simulink library "SUB_ECU_L4_MABX_HW_Interface_PIC_KW"  (R2018a)
settings: Solver=VariableStepAuto  StartTime=0.0  StopTime=10.0  RelTol=1e-3
PostLoadFcn:
  | , if any(exist('dsrtsu_mdlpostloadfcn', 'file') == [2, 3, 6]), try dsrtsu_mdlpostloadfcn('Execute', bdroot); catch fprintf('Error in PostLoadFcn (dsrtsu_mdlpostloadfcn) for model "%s":\n %s\n', bdroot, lasterr); end, end,
undefined symbols (not defined in the file or in its folder): CANR_PROPB_REAX_3_13_CHANNEL_APV, CANR_PROPB_REAX_4_13_CHANNEL_APV, CANR_PROPB_XPR_1_50_CHANNEL_APV, ENUM_CAN_RX_T, ENUM_CAN_TX_T, ENUM_REAX_OPERATION_MODE_T, ENUM_SIGNAL_HEALTH_T, ENUM_XBR_CONTROL_MODE_T, ENUM_XBR_EBI_MODE_T, ENUM_XBR_PASS_THROUGH_ACTIVE_T, ENUM_XBR_PRIORITY_T, ENUM_XPR_INHIBIT_PARK_MANUAL_T, ENUM_XPR_INHIBIT_UNPARK_MANUAL_T, ENUM_XPR_PARK_MANUAL_T, ENUM_XPR_UNPARK_MANUAL_T, PROPB_REAX_1_E4_DES_POS_SIG_SRC_APV, PROPB_REAX_1_E4_DESIRED_OPMODE_APV, PROPB_REAX_1_E4_DESIRED_POSITION_APV, PROPB_REAX_CHANNEL_APV, ptc_matlab_lib
libraries: PTC_MBDS_LIB x292, rtican x158, simulink x58, EmE_MBD_Blockset x38, rti1401lib_dio_type4 x13, simulink_need_slupdate x7, rti1401lib_adc_type4 x3, rtmapslib x3, $bdroot x3, dsa_tcpip_lib x2, SUB_ECU_L4_MABX_HW_Interface_PTC_1571 x1, rtitasklib x1
(part 13 of 48)

== system SUB_ECU_L4_MABX_HW_Interface_PIC_KW/CAN_PIC_KW/CAN_RX_EEC1_00/RX_CAN_1 ==
  Enable : Inport
  Bus Creator3 : BusCreator  Inputs=11
  Data Type Conversion10 : DataTypeConversion  OutDataTypeStr=double  SaturateOnIntegerOverflow=on
  Data Type Conversion8 : DataTypeConversion  OutDataTypeStr=boolean  SaturateOnIntegerOverflow=on
  Data Type Conversion9 : DataTypeConversion  OutDataTypeStr=double  SaturateOnIntegerOverflow=on
  EEC1_001 : rtican/RTICAN Receive (RX)   Reserved1=[]  Reserved2=[]  Reserved3=[]  Reserved4=[]  SfcnMessage=[]  Msg_Struct=[]  BoardTypeNo=[]  BoardNo=[]  ChannelNo=[]  Parameters=[]  DialogFcn=[]  UnitName=[]  Revision=[]  UnitValues=[]  DSProperties=struct('RTI',struct('Version',uint32(5),'BlockType',struct('isSLSource',uint8(1),'isSLSink',uint8(1),'isHWSource',uint8(0),'isHWSink',uint8(0),'isSetup',uint8(0),'isInline',uint8(1),'isNonInline',uint8(0),'isInterrupt',uint8(0),'isChannelwise',uint8(0)),'IOBoardType','RTICAN','UnitType','MESSAGE','Identifier','RX','DialogType','MSVC','BlockSet','RTICAN','SlaveProcessor','CAN'))  RTIBlockInterface=struct('OutputPortsWidth',int32([1 1 1 1 1 1 1 1 1 1 1]),'OutputPortsActive',ones(1,11),'OutputPortsName',{{'EngTorqueMode','ActlEngPrcntTrqueHighResolution','DriversDemandEngPercentTorque','ActualEngPercentTorque','EngSpeed','SrcAddrssOfCtrllngDvcFrEngCntrl','EngStarterMode','EngDemandPercentTorque',['RX status'],['RX time'],['RX delta time']}},'OutputPortsDataType',{{'SS_DOUBLE','SS_DOUBLE','SS_DOUBLE','SS_DOUBLE','SS_DOUBLE','SS_DOUBLE','SS_DOUBLE','SS_DOUBLE','SS_DOUBLE','SS_DOUBLE','SS_DOUBLE'}},'OutputPortsLabel',{{'EngTorqueMode','ActlEngPrcntTrqueHighResolution','DriversDemandEngPercentTorque','ActualEngPercentTorque','EngSpeed','SrcAddrssOfCtrllngDvcFrEngCntrl','EngStarterMode','EngDemandPercentTorque','','',''}},'OutputPortsLabelMode','ON','InputPortsWidth',int32(0),'InputPortsActive',0,'DialogFcn','rtican_message_interface_gui','BlockDisplay',{{'','center'}},'IconTransparency','on','ParameterTunableNames',{{}},'InitLevel',3,'BlockName',struct('Token',{{'EEC1_00'}}),'SampleTime',{{-1}},'TriggerPort',{{'none'}},'EnablePort',{{'yes'}})  RTIBlockParameters=struct('BoardTypeNo',{{1,'OFF',[]}},'BoardNo',{{1,'ON',[1 16]}},'ChannelNo',{{1,'ON',[1 2]}},'Parameters',{{struct('DataFileSupport',struct('DataFileSelectedMaster',1,'DataFileSelectedLocal',1,'DataFileName','c:\localdata\chris\advanced_tech\adas\level4_rcp\truck1571\dbc\j1939_famosdbcwithfusion.dbc|','DataFileDate',{{{['03-Apr-2017 12:55:40']}}},'SelectedFile','dbc\j1939_famosdbcwithfusion.dbc'),'Options',struct('StatusSelected',1,'TimeSelected',1,'DeltaTimeSelected',1,'BytePortSelected',0,'MessageLengthSelected',0,'TriggerPort',struct('Selected',0,'TriggerType',0),'UserCoding',struct('Selected',0,'InterfaceFile','UserDecodingFile','FcnName','UserDecodeFcn','InportSelected',0,'InportWidth',1,'OutportSelected',0,'OutportWidth',1),'EnablePortSelected',1,'SignalOnPortnameSelected',1,'UseRXService',1),'Message',struct('MsgOnBlocknameSelected',1,'MsgName','EEC1_00','MsgIdFormat',1,'MsgId',217056256,'MsgLength',8,'NumSignals',8,'SampleTime',-1,'Signal',struct('SgnName',{'EngTorqueMode','ActlEngPrcntTrqueHighResolution','DriversDemandEngPercentTorque','ActualEngPercentTorque','EngSpeed','SrcAddrssOfCtrllngDvcFrEngCntrl','EngStarterMode','EngDemandPercentTorque'},'SgnStartBit',{0,4,8,16,24,40,48,56},'SgnLength',{4,4,8,8,16,8,4,8},'SgnType',{0,0,0,0,0,0,0,0},'ModeValue',{-1,-1,-1,-1,-1,-1,-1,-1},'DataType',{0,0,0,0,0,0,0,0},'ByteLayout',{0,0,0,0,0,0,0,0},'Factor',{1,2^-3,1,1,2^-3,1,1,1},'Offset',{0,0,-125,-125,0,0,0,-125},'SgnComment',{{['State signal which indicates which engine torque mode is currently generating, limiting, or controlling the torque.']},{['This parameter displays an additional torque in percent of the reference engine torque.']},{['The requested torque output of the engine by the driver.']},{['The calculated output torque of the engine.']},{['Actual engine speed which is calculated over a minimum crankshaft angle of 720 degrees divided by the number of cylinders.']},{['The source address of the SAE J1939 device currently controlling the engine.']},{['There are several phases in a starting action and different reasons why a start cannot take place.']},{['The requested torque output of the engine by all dynamic internal inputs, including smoke control, noise control and low']}},'SgnUnit',{'','%','%','%','rpm','','','%'},'Min',{0,0,-125,-125,0,0,0,-125},'Max',{15,0.875,125,125,8031.875,255,15,125},'SLDataType',{'SS_DOUBLE','SS_DOUBLE','SS_DOUBLE','SS_DOUBLE','SS_DOUBLE','SS_DOUBLE','SS_DOUBLE','SS_DOUBLE'}),'MsgIdNumFormat',0,'MsgComment',{{['Electronic Engine Controller 1']}}),'Version',1.2,'general',struct('isFromLib',0)),'OFF',[]}},'GroupId',{{struct('Group',{{'RTICAN'}},'No',1,'Behavior',{{'NAMECHANGE'}},'BlockType',{{'SINK'}},'NameChangeFlag',0),'OFF',[]}},'SFcnRTICANMessage',{{struct('MsgType','RX','SFcnPortType','Scalar','MsgName','EEC1_00','MsgIdFormat','XTD','MsgId',217056256,'MsgLength',8,'NumSignals',8,'SampleTime',-1,'Signal',struct('SgnName',{'EngTorqueMode','ActlEngPrcntTrqueHighResolution','DriversDemandEngPercentTorque','ActualEngPercentTorque','EngSpeed','SrcAddrssOfCtrllngDvcFrEngCntrl','EngStarterMode','EngDemandPercentTorque'},'SgnStartBit',{0,4,8,16,24,40,48,56},'SgnLength',{4,4,8,8,16,8,4,8},'SgnType',{'standard','standard','standard','standard','standard','standard','standard','standard'},'ModeValue',{-1,-1,-1,-1,-1,-1,-1,-1},'DataType',{['unsigned int'],['unsigned int'],['unsigned int'],['unsigned int'],['unsigned int'],['unsigned int'],['unsigned int'],['unsigned int']},'ByteLayout',{['little endian'],['little endian'],['little endian'],['little endian'],['little endian'],['little endian'],['little endian'],['little endian']},'Factor',{1,2^-3,1,1,2^-3,1,1,1},'Offset',{0,0,-125,-125,0,0,0,-125},'SLDataType',{'SS_DOUBLE','SS_DOUBLE','SS_DOUBLE','SS_DOUBLE','SS_DOUBLE','SS_DOUBLE','SS_DOUBLE','SS_DOUBLE'}),'StatusSelected','yes','TimeSelected','yes','DeltaTimeSelected','yes','BytePortSelected','no','MessageLengthSelected','no','TriggerPort',struct('Selected','no','TriggerType',0),'UserCoding',struct('Selected','no','InterfaceFile','UserDecodingFile','FcnName','UserDecodeFcn','InportSelected','no','InportWidth',1,'OutportSelected','no','OutportWidth',1),'EnablePortSelected','yes','UseRXService','yes','BoardType','DS1','BoardNo',1,'ControllerNo',1),'OFF',[]}},'TLCFileName',{{'rtican_rx_message','OFF',[]}})  RTISFcnParameters=struct('SFcnRTICANMessage','struct','TLCFileName','char')  RTIBlockParaDefault=struct('BoardTypeNo',4302,'BoardNo',1,'ChannelNo',1,'Parameters',struct('DataFileSupport',struct('DataFileSelectedMaster',0,'DataFileSelectedLocal',0,'DataFileName','','DataFileDate','','SelectedFile',['<no file selected>']),'Options',struct('StatusSelected',1,'TimeSelected',1,'DeltaTimeSelected',1,'BytePortSelected',0,'MessageLengthSelected',0,'TriggerPort',struct('Selected',0,'TriggerType','rising'),'UserCoding',struct('Selected',0,'InterfaceFile','UserDecodingFile','FcnName','UserDecodeFcn','InportSelected',0,'InportWidth',1,'OutportSelected',0,'OutportWidth',1),'EnablePortSelected',0,'SignalOnPortnameSelected',1,'UseRXService',0),'Message',struct('MsgOnBlocknameSelected',0,'MsgName',['RX Message'],'MsgIdFormat',0,'MsgId',100,'MsgLength',8,'NumSignals',1,'SampleTime',-1,'Signal',struct('SgnName',['RX signal'],'SgnStartBit',0,'SgnLength',8,'SgnType',0,'ModeValue',-1,'DataType',0,'SLDataType','SS_DOUBLE','ByteLayout',0,'Factor',1,'Offset',0,'Min',0,'Max',255,'SgnComment',{{}},'SgnUnit',''),'MsgIdNumFormat',0,'MsgComment',{{''}}),'Version',1.2,'general',struct('isFromLib',1)),'GroupId',struct('Group',{{'RTICAN'}},'No',1,'Behavior',{{'NAMECHANGE'}},'BlockType',{{'SINK'}},'NameChangeFlag',0),'SFcnRTICANMessage',struct('MsgType','RX','MsgName',['RX Message'],'MsgIdFormat','STD','MsgId',100,'MsgLength',8,'NumSignals',1,'SampleTime',-1,'Signal',struct('SgnName',['RX signal'],'SgnStartBit',0,'SgnLength',8,'SgnType','standard','ModeValue',-1,'DataType',['unsigned int'],'ByteLayout',['little endian'],'SLDataType','SS_DOUBLE','Factor',1,'Offset',0),'StatusSelected','yes','TimeSelected','yes','DeltaTimeSelected','yes','BytePortSelected','no','MessageLengthSelected','no','EnablePortSelected','no','UserCoding',struct('Selected','no','InterfaceFile','UserDecodingFile','FcnName','UserDecodeFcn','InportSelected','no','InportWidth',1,'OutportSelected','no','OutportWidth',1),'TriggerPort',struct('Selected','no','TriggerType','rising'),'UseRXService','no','BoardType','DS4302','BoardNo',1,'ControllerNo',1,'SFcnPortType','Scalar'),'TLCFileName','rtican_rx_message')
      settings: AttributesFormatString=Group Id: RTICAN1\n  SourceProductName=dSPACE RTI CAN Blockset
  EEC1_00 : Outport
  wires:
  Bus Creator3/1 -> EEC1_00/1  "EEC1_00"
  EEC1_001/11 -> Data Type Conversion10/1
  EEC1_001/10 -> Data Type Conversion9/1
  EEC1_001/9 -> Data Type Conversion8/1
  Enable/1 -> EEC1_001/Enable
  Data Type Conversion8/1 -> Bus Creator3/9  "RX_status"
  Data Type Conversion10/1 -> Bus Creator3/11  "RX_delta_time"
  Data Type Conversion9/1 -> Bus Creator3/10  "RX_time"
  EEC1_001/6 -> Bus Creator3/6  "SrcAddrssOfCtrllngDvcFrEngCntrl"
  EEC1_001/4 -> Bus Creator3/4  "ActualEngPercentTorque"
  EEC1_001/7 -> Bus Creator3/7  "EngStarterMode"
  EEC1_001/1 -> Bus Creator3/1  "EngTorqueMode"
  EEC1_001/2 -> Bus Creator3/2  "ActlEngPrcntTrqueHighResolution"
  EEC1_001/8 -> Bus Creator3/8  "EngDemandPercentTorque"
  EEC1_001/5 -> Bus Creator3/5  "EngSpeed"
  EEC1_001/3 -> Bus Creator3/3  "DriversDemandEngPercentTorque"

== system SUB_ECU_L4_MABX_HW_Interface_PIC_KW/CAN_PIC_KW/CAN_RX_EEC2_00/RX_CAN_2 ==
  Enable : Inport
  Bus Creator3 : BusCreator  Inputs=17
  Data Type Conversion10 : DataTypeConversion  OutDataTypeStr=double  SaturateOnIntegerOverflow=on
  Data Type Conversion8 : DataTypeConversion  OutDataTypeStr=boolean  SaturateOnIntegerOverflow=on
  Data Type Conversion9 : DataTypeConversion  OutDataTypeStr=double  SaturateOnIntegerOverflow=on
  EEC2_001 : rtican/RTICAN Receive (RX)   Reserved1=[]  Reserved2=[]  Reserved3=[]  Reserved4=[]  SfcnMessage=[]  Msg_Struct=[]  BoardTypeNo=[]  BoardNo=[]  ChannelNo=[]  Parameters=[]  DialogFcn=[]  UnitName=[]  Revision=[]  UnitValues=[]  DSProperties=struct('RTI',struct('Version',uint32(5),'BlockType',struct('isSLSource',uint8(1),'isSLSink',uint8(1),'isHWSource',uint8(0),'isHWSink',uint8(0),'isSetup',uint8(0),'isInline',uint8(1),'isNonInline',uint8(0),'isInterrupt',uint8(0),'isChannelwise',uint8(0)),'IOBoardType','RTICAN','UnitType','MESSAGE','Identifier','RX','DialogType','MSVC','BlockSet','RTICAN','SlaveProcessor','CAN'))  RTIBlockInterface=struct('OutputPortsWidth',int32([1 1 1 1 1 1 1 1 1 1 1 1 1 1 1 1 1]),'OutputPortsActive',ones(1,17),'OutputPortsName',{{'SPN558_AccelPed1LowIdlSwitch','SPN559_AccelPedKickdownSw','SPN1437_RoadSpeedLimitStatus','SPN2970_AccelPed2LowIdlSwitch','SPN91_AccelPedPos1','SPN92_EngPercLoadAtCurrSpd','SPN974_RemAccelPedalPosition','SPN29_AccelPedPos2','SPN2979_VehAccelRateLimStatus','SPN5021_MomEngMaxPwrEnFdbk','SPN5399_DPFThermMgmtActive','SPN5400_SCRThermMgmtActive','SPN3357_ActMaxAvailEngPercTrq','SPN5398_EstPumpingPercentTorque',['RX status'],['RX time'],['RX delta time']}},'OutputPortsDataType',{{'SS_DOUBLE','SS_DOUBLE','SS_DOUBLE','SS_DOUBLE','SS_DOUBLE','SS_DOUBLE','SS_DOUBLE','SS_DOUBLE','SS_DOUBLE','SS_DOUBLE','SS_DOUBLE','SS_DOUBLE','SS_DOUBLE','SS_DOUBLE','SS_DOUBLE','SS_DOUBLE','SS_DOUBLE'}},'OutputPortsLabel',{{'SPN558_AccelPed1LowIdlSwitch','SPN559_AccelPedKickdownSw','SPN1437_RoadSpeedLimitStatus','SPN2970_AccelPed2LowIdlSwitch','SPN91_AccelPedPos1','SPN92_EngPercLoadAtCurrSpd','SPN974_RemAccelPedalPosition','SPN29_AccelPedPos2','SPN2979_VehAccelRateLimStatus','SPN5021_MomEngMaxPwrEnFdbk','SPN5399_DPFThermMgmtActive','SPN5400_SCRThermMgmtActive','SPN3357_ActMaxAvailEngPercTrq','SPN5398_EstPumpingPercentTorque','','',''}},'OutputPortsLabelMode','ON','InputPortsWidth',int32(0),'InputPortsActive',0,'DialogFcn','rtican_message_interface_gui','BlockDisplay',{{'','center'}},'IconTransparency','on','ParameterTunableNames',{{}},'InitLevel',3,'BlockName',struct('Token',{{'EEC2_00'}}),'SampleTime',{{-1}},'TriggerPort',{{'none'}},'EnablePort',{{'yes'}})  RTIBlockParameters=struct('BoardTypeNo',{{1,'OFF',[]}},'BoardNo',{{1,'ON',[1 16]}},'ChannelNo',{{2,'ON',[1 2]}},'Parameters',{{struct('DataFileSupport',struct('DataFileSelectedMaster',1,'DataFileSelectedLocal',0,'DataFileName','i:\435\team\balton\truck1571\dbc\mabx_can2.dbc|','DataFileDate',{{{['01-Feb-2017 13:05:11']}}},'SelectedFile',['<no file selected>']),'Options',struct('StatusSelected',1,'TimeSelected',1,'DeltaTimeSelected',1,'BytePortSelected',0,'MessageLengthSelected',0,'TriggerPort',struct('Selected',0,'TriggerType',0),'UserCoding',struct('Selected',0,'InterfaceFile','UserDecodingFile','FcnName','UserDecodeFcn','InportSelected',0,'InportWidth',1,'OutportSelected',0,'OutportWidth',1),'EnablePortSelected',1,'SignalOnPortnameSelected',1,'UseRXService',1),'Message',struct('MsgOnBlocknameSelected',1,'MsgName','EEC2_00','MsgIdFormat',1,'MsgId',217056000,'MsgLength',8,'NumSignals',14,'SampleTime',-1,'Signal',struct('SgnName',{'SPN558_AccelPed1LowIdlSwitch','SPN559_AccelPedKickdownSw','SPN1437_RoadSpeedLimitStatus','SPN2970_AccelPed2LowIdlSwitch','SPN91_AccelPedPos1','SPN92_EngPercLoadAtCurrSpd','SPN974_RemAccelPedalPosition','SPN29_AccelPedPos2','SPN2979_VehAccelRateLimStatus','SPN5021_MomEngMaxPwrEnFdbk','SPN5399_DPFThermMgmtActive','SPN5400_SCRThermMgmtActive','SPN3357_ActMaxAvailEngPercTrq','SPN5398_EstPumpingPercentTorque'},'SgnStartBit',{0,2,4,6,8,16,24,32,40,42,44,46,48,56},'SgnLength',{2,2,2,2,8,8,8,8,2,2,2,2,8,8},'SgnType',{0,0,0,0,0,0,0,0,0,0,0,0,0,0},'ModeValue',{-1,-1,-1,-1,-1,-1,-1,-1,-1,-1,-1,-1,-1,-1},'DataType',{0,0,0,0,0,0,0,0,0,0,0,0,0,0},'ByteLayout',{0,0,0,0,0,0,0,0,0,0,0,0,0,0},'Factor',{1,1,1,1,0.4,1,0.4,0.4,1,1,1,1,0.4,1},'Offset',{0,0,0,0,0,0,0,0,0,0,0,0,0,-125},'SgnComment',{{['Accelerator Pedal 1 Low Idle Switch']},{['Accelerator Pedal Kickdown Switch']},{['Road Speed Limit Status']},{['Accelerator Pedal 2 Low Idle Switch']},{['Accelerator Pedal Position 1']},{['Engine Percent Load At Current Speed']},{['Remote Accelerator Pedal Position']},{['Accelerator Pedal Position 2']},{['Vehicle Acceleration Rate Limit Status']},{['Momentary Engine Maximum Power Enable Feedback']},{['DPF Thermal Management Active']},{['SCR Thermal Management Active']},{['Actual Maximum Available Engine - Percent Torque']},{['Estimated Pumping - Percent Torque']}},'SgnUnit',{'bit','bit','bit','bit','%','%','%','%','bit','bit','bit','bit','%','%'},'Min',{0,0,0,0,0,0,0,0,0,0,0,0,0,-125},'Max',{3,3,3,3,100,250,100,100,3,3,3,3,100,125},'SLDataType',{'SS_DOUBLE','SS_DOUBLE','SS_DOUBLE','SS_DOUBLE','SS_DOUBLE','SS_DOUBLE','SS_DOUBLE','SS_DOUBLE','SS_DOUBLE','SS_DOUBLE','SS_DOUBLE','SS_DOUBLE','SS_DOUBLE','SS_DOUBLE'}),'MsgIdNumFormat',0,'MsgComment',{{['Electronic Engine Controller 2']}}),'Version',1.2,'general',struct('isFromLib',0)),'OFF',[]}},'GroupId',{{struct('Group',{{'RTICAN'}},'No',2,'Behavior',{{'NAMECHANGE'}},'BlockType',{{'SINK'}},'NameChangeFlag',0),'OFF',[]}},'SFcnRTICANMessage',{{struct('MsgType','RX','SFcnPortType','Scalar','MsgName','EEC2_00','MsgIdFormat','XTD','MsgId',217056000,'MsgLength',8,'NumSignals',14,'SampleTime',-1,'Signal',struct('SgnName',{'SPN558_AccelPed1LowIdlSwitch','SPN559_AccelPedKickdownSw','SPN1437_RoadSpeedLimitStatus','SPN2970_AccelPed2LowIdlSwitch','SPN91_AccelPedPos1','SPN92_EngPercLoadAtCurrSpd','SPN974_RemAccelPedalPosition','SPN29_AccelPedPos2','SPN2979_VehAccelRateLimStatus','SPN5021_MomEngMaxPwrEnFdbk','SPN5399_DPFThermMgmtActive','SPN5400_SCRThermMgmtActive','SPN3357_ActMaxAvailEngPercTrq','SPN5398_EstPumpingPercentTorque'},'SgnStartBit',{0,2,4,6,8,16,24,32,40,42,44,46,48,56},'SgnLength',{2,2,2,2,8,8,8,8,2,2,2,2,8,8},'SgnType',{'standard','standard','standard','standard','standard','standard','standard','standard','standard','standard','standard','standard','standard','standard'},'ModeValue',{-1,-1,-1,-1,-1,-1,-1,-1,-1,-1,-1,-1,-1,-1},'DataType',{['unsigned int'],['unsigned int'],['unsigned int'],['unsigned int'],['unsigned int'],['unsigned int'],['unsigned int'],['unsigned int'],['unsigned int'],['unsigned int'],['unsigned int'],['unsigned int'],['unsigned int'],['unsigned int']},'ByteLayout',{['little endian'],['little endian'],['little endian'],['little endian'],['little endian'],['little endian'],['little endian'],['little endian'],['little endian'],['little endian'],['little endian'],['little endian'],['little endian'],['little endian']},'Factor',{1,1,1,1,0.4,1,0.4,0.4,1,1,1,1,0.4,1},'Offset',{0,0,0,0,0,0,0,0,0,0,0,0,0,-125},'SLDataType',{'SS_DOUBLE','SS_DOUBLE','SS_DOUBLE','SS_DOUBLE','SS_DOUBLE','SS_DOUBLE','SS_DOUBLE','SS_DOUBLE','SS_DOUBLE','SS_DOUBLE','SS_DOUBLE','SS_DOUBLE','SS_DOUBLE','SS_DOUBLE'}),'StatusSelected','yes','TimeSelected','yes','DeltaTimeSelected','yes','BytePortSelected','no','MessageLengthSelected','no','TriggerPort',struct('Selected','no','TriggerType',0),'UserCoding',struct('Selected','no','InterfaceFile','UserDecodingFile','FcnName','UserDecodeFcn','InportSelected','no','InportWidth',1,'OutportSelected','no','OutportWidth',1),'EnablePortSelected','yes','UseRXService','yes','BoardType','DS1','BoardNo',1,'ControllerNo',1),'OFF',[]}},'TLCFileName',{{'rtican_rx_message','OFF',[]}})  RTISFcnParameters=struct('SFcnRTICANMessage','struct','TLCFileName','char')  RTIBlockParaDefault=struct('BoardTypeNo',4302,'BoardNo',1,'ChannelNo',1,'Parameters',struct('DataFileSupport',struct('DataFileSelectedMaster',0,'DataFileSelectedLocal',0,'DataFileName','','DataFileDate','','SelectedFile',['<no file selected>']),'Options',struct('StatusSelected',1,'TimeSelected',1,'DeltaTimeSelected',1,'BytePortSelected',0,'MessageLengthSelected',0,'TriggerPort',struct('Selected',0,'TriggerType','rising'),'UserCoding',struct('Selected',0,'InterfaceFile','UserDecodingFile','FcnName','UserDecodeFcn','InportSelected',0,'InportWidth',1,'OutportSelected',0,'OutportWidth',1),'EnablePortSelected',0,'SignalOnPortnameSelected',1,'UseRXService',0),'Message',struct('MsgOnBlocknameSelected',0,'MsgName',['RX Message'],'MsgIdFormat',0,'MsgId',100,'MsgLength',8,'NumSignals',1,'SampleTime',-1,'Signal',struct('SgnName',['RX signal'],'SgnStartBit',0,'SgnLength',8,'SgnType',0,'ModeValue',-1,'DataType',0,'SLDataType','SS_DOUBLE','ByteLayout',0,'Factor',1,'Offset',0,'Min',0,'Max',255,'SgnComment',{{}},'SgnUnit',''),'MsgIdNumFormat',0,'MsgComment',{{''}}),'Version',1.2,'general',struct('isFromLib',1)),'GroupId',struct('Group',{{'RTICAN'}},'No',1,'Behavior',{{'NAMECHANGE'}},'BlockType',{{'SINK'}},'NameChangeFlag',0),'SFcnRTICANMessage',struct('MsgType','RX','MsgName',['RX Message'],'MsgIdFormat','STD','MsgId',100,'MsgLength',8,'NumSignals',1,'SampleTime',-1,'Signal',struct('SgnName',['RX signal'],'SgnStartBit',0,'SgnLength',8,'SgnType','standard','ModeValue',-1,'DataType',['unsigned int'],'ByteLayout',['little endian'],'SLDataType','SS_DOUBLE','Factor',1,'Offset',0),'StatusSelected','yes','TimeSelected','yes','DeltaTimeSelected','yes','BytePortSelected','no','MessageLengthSelected','no','EnablePortSelected','no','UserCoding',struct('Selected','no','InterfaceFile','UserDecodingFile','FcnName','UserDecodeFcn','InportSelected','no','InportWidth',1,'OutportSelected','no','OutportWidth',1),'TriggerPort',struct('Selected','no','TriggerType','rising'),'UseRXService','no','BoardType','DS4302','BoardNo',1,'ControllerNo',1,'SFcnPortType','Scalar'),'TLCFileName','rtican_rx_message')
      settings: AttributesFormatString=Group Id: RTICAN2\n  SourceProductName=dSPACE RTI CAN Blockset
  EEC2_00 : Outport
  wires:
  Bus Creator3/1 -> EEC2_00/1  "EEC2_00"
  Enable/1 -> EEC2_001/Enable
  EEC2_001/17 -> Data Type Conversion10/1
  EEC2_001/16 -> Data Type Conversion9/1
  EEC2_001/15 -> Data Type Conversion8/1
  Data Type Conversion8/1 -> Bus Creator3/15  "RX_status"
  Data Type Conversion10/1 -> Bus Creator3/17  "RX_delta_time"
  Data Type Conversion9/1 -> Bus Creator3/16  "RX_time"
  EEC2_001/11 -> Bus Creator3/11  "SPN5399_DPFThermMgmtActive"
  EEC2_001/14 -> Bus Creator3/14  "SPN5398_EstPumpingPercentTorque"
  EEC2_001/12 -> Bus Creator3/12  "SPN5400_SCRThermMgmtActive"
  EEC2_001/13 -> Bus Creator3/13  "SPN3357_ActMaxAvailEngPercTrq"
  EEC2_001/10 -> Bus Creator3/10  "SPN5021_MomEngMaxPwrEnFdbk"
  EEC2_001/1 -> Bus Creator3/1  "SPN558_AccelPed1LowIdlSwitch"
  EEC2_001/2 -> Bus Creator3/2  "SPN559_AccelPedKickdownSw"
  EEC2_001/5 -> Bus Creator3/5  "SPN91_AccelPedPos1"
  EEC2_001/6 -> Bus Creator3/6  "SPN92_EngPercLoadAtCurrSpd"
  EEC2_001/8 -> Bus Creator3/8  "SPN29_AccelPedPos2"
  EEC2_001/9 -> Bus Creator3/9  "SPN2979_VehAccelRateLimStatus"
  EEC2_001/3 -> Bus Creator3/3  "SPN1437_RoadSpeedLimitStatus"
  EEC2_001/4 -> Bus Creator3/4  "SPN2970_AccelPed2LowIdlSwitch"
  EEC2_001/7 -> Bus Creator3/7  "SPN974_RemAccelPedalPosition"

== system SUB_ECU_L4_MABX_HW_Interface_PIC_KW/CAN_PIC_KW/CAN_RX_EEC3_00/RX_CAN_1 ==
  Enable : Inport
  Bus Creator3 : BusCreator  Inputs=5
  Data Type Conversion{1..2,9..10} (4 alike) : DataTypeConversion  OutDataTypeStr=double  SaturateOnIntegerOverflow=on
  Data Type Conversion8 : DataTypeConversion  OutDataTypeStr=boolean  SaturateOnIntegerOverflow=on
  EEC3_001 : rtican/RTICAN Receive (RX)   Reserved1=[]  Reserved2=[]  Reserved3=[]  Reserved4=[]  SfcnMessage=[]  Msg_Struct=[]  BoardTypeNo=[]  BoardNo=[]  ChannelNo=[]  Parameters=[]  DialogFcn=[]  UnitName=[]  Revision=[]  UnitValues=[]  DSProperties=struct('RTI',struct('Version',uint32(5),'BlockType',struct('isSLSource',uint8(1),'isSLSink',uint8(1),'isHWSource',uint8(0),'isHWSink',uint8(0),'isSetup',uint8(0),'isInline',uint8(1),'isNonInline',uint8(0),'isInterrupt',uint8(0),'isChannelwise',uint8(0)),'IOBoardType','RTICAN','UnitType','MESSAGE','Identifier','RX','DialogType','MSVC','BlockSet','RTICAN','SlaveProcessor','CAN'))  RTIBlockInterface=struct('OutputPortsWidth',int32([1 1 1 1 1]),'OutputPortsActive',[1 1 1 1 1],'OutputPortsName',{{'SPN514_NominalFrictionPercentTorque','SPN2978_EstEngParasiticLossesPercentTorque',['RX status'],['RX time'],['RX delta time']}},'OutputPortsDataType',{{'SS_DOUBLE','SS_DOUBLE','SS_DOUBLE','SS_DOUBLE','SS_DOUBLE'}},'OutputPortsLabel',{{'SPN514_NominalFrictionPercentTorque','SPN2978_EstEngParasiticLossesPercentTorque','','',''}},'OutputPortsLabelMode','ON','InputPortsWidth',int32(0),'InputPortsActive',0,'DialogFcn','rtican_message_interface_gui','BlockDisplay',{{'','center'}},'IconTransparency','on','ParameterTunableNames',{{}},'InitLevel',3,'BlockName',struct('Token',{{'EEC3_00'}}),'SampleTime',{{-1}},'TriggerPort',{{'none'}},'EnablePort',{{'yes'}})  RTIBlockParameters=struct('BoardTypeNo',{{1,'OFF',[]}},'BoardNo',{{1,'ON',[1 16]}},'ChannelNo',{{1,'ON',[1 2]}},'Parameters',{{struct('DataFileSupport',struct('DataFileSelectedMaster',1,'DataFileSelectedLocal',0,'DataFileName','i:\435\team\balton\truck1571\dbc\mabx_can1.dbc|','DataFileDate',{{{['01-Feb-2017 13:05:11']}}},'SelectedFile',['<no file selected>']),'Options',struct('StatusSelected',1,'TimeSelected',1,'DeltaTimeSelected',1,'BytePortSelected',0,'MessageLengthSelected',0,'TriggerPort',struct('Selected',0,'TriggerType',0),'UserCoding',struct('Selected',0,'InterfaceFile','UserDecodingFile','FcnName','UserDecodeFcn','InportSelected',0,'InportWidth',1,'OutportSelected',0,'OutportWidth',1),'EnablePortSelected',1,'SignalOnPortnameSelected',1,'UseRXService',1),'Message',struct('MsgOnBlocknameSelected',1,'MsgName','EEC3_00','MsgIdFormat',1,'MsgId',419356416,'MsgLength',8,'NumSignals',2,'SampleTime',-1,'Signal',struct('SgnName',{'SPN514_NominalFrictionPercentTorque','SPN2978_EstEngParasiticLossesPercentTorque'},'SgnStartBit',{0,32},'SgnLength',{8,8},'SgnType',{0,0},'ModeValue',{-1,-1},'DataType',{0,0},'ByteLayout',{0,0},'Factor',{1,1},'Offset',{-125,-125},'SgnComment',{{['SCR Thermal Management Active']},{['SCR Thermal Management Active']}},'SgnUnit',{'%','%'},'Min',{0,0},'Max',{3,3},'SLDataType',{'SS_DOUBLE','SS_DOUBLE'}),'MsgIdNumFormat',1,'MsgComment',{{['Electronic Engine Controller 3']}}),'Version',1.2,'general',struct('isFromLib',0)),'OFF',[]}},'GroupId',{{struct('Group',{{'RTICAN'}},'No',1,'Behavior',{{'NAMECHANGE'}},'BlockType',{{'SINK'}},'NameChangeFlag',0),'OFF',[]}},'SFcnRTICANMessage',{{struct('MsgType','RX','SFcnPortType','Scalar','MsgName','EEC3_00','MsgIdFormat','XTD','MsgId',419356416,'MsgLength',8,'NumSignals',2,'SampleTime',-1,'Signal',struct('SgnName',{'SPN514_NominalFrictionPercentTorque','SPN2978_EstEngParasiticLossesPercentTorque'},'SgnStartBit',{0,32},'SgnLength',{8,8},'SgnType',{'standard','standard'},'ModeValue',{-1,-1},'DataType',{['unsigned int'],['unsigned int']},'ByteLayout',{['little endian'],['little endian']},'Factor',{1,1},'Offset',{-125,-125},'SLDataType',{'SS_DOUBLE','SS_DOUBLE'}),'StatusSelected','yes','TimeSelected','yes','DeltaTimeSelected','yes','BytePortSelected','no','MessageLengthSelected','no','TriggerPort',struct('Selected','no','TriggerType',0),'UserCoding',struct('Selected','no','InterfaceFile','UserDecodingFile','FcnName','UserDecodeFcn','InportSelected','no','InportWidth',1,'OutportSelected','no','OutportWidth',1),'EnablePortSelected','yes','UseRXService','yes','BoardType','DS1','BoardNo',1,'ControllerNo',2),'OFF',[]}},'TLCFileName',{{'rtican_rx_message','OFF',[]}})  RTISFcnParameters=struct('SFcnRTICANMessage','struct','TLCFileName','char')  RTIBlockParaDefault=struct('BoardTypeNo',4302,'BoardNo',1,'ChannelNo',1,'Parameters',struct('DataFileSupport',struct('DataFileSelectedMaster',0,'DataFileSelectedLocal',0,'DataFileName','','DataFileDate','','SelectedFile',['<no file selected>']),'Options',struct('StatusSelected',1,'TimeSelected',1,'DeltaTimeSelected',1,'BytePortSelected',0,'MessageLengthSelected',0,'TriggerPort',struct('Selected',0,'TriggerType','rising'),'UserCoding',struct('Selected',0,'InterfaceFile','UserDecodingFile','FcnName','UserDecodeFcn','InportSelected',0,'InportWidth',1,'OutportSelected',0,'OutportWidth',1),'EnablePortSelected',0,'SignalOnPortnameSelected',1,'UseRXService',0),'Message',struct('MsgOnBlocknameSelected',0,'MsgName',['RX Message'],'MsgIdFormat',0,'MsgId',100,'MsgLength',8,'NumSignals',1,'SampleTime',-1,'Signal',struct('SgnName',['RX signal'],'SgnStartBit',0,'SgnLength',8,'SgnType',0,'ModeValue',-1,'DataType',0,'SLDataType','SS_DOUBLE','ByteLayout',0,'Factor',1,'Offset',0,'Min',0,'Max',255,'SgnComment',{{}},'SgnUnit',''),'MsgIdNumFormat',0,'MsgComment',{{''}}),'Version',1.2,'general',struct('isFromLib',1)),'GroupId',struct('Group',{{'RTICAN'}},'No',1,'Behavior',{{'NAMECHANGE'}},'BlockType',{{'SINK'}},'NameChangeFlag',0),'SFcnRTICANMessage',struct('MsgType','RX','MsgName',['RX Message'],'MsgIdFormat','STD','MsgId',100,'MsgLength',8,'NumSignals',1,'SampleTime',-1,'Signal',struct('SgnName',['RX signal'],'SgnStartBit',0,'SgnLength',8,'SgnType','standard','ModeValue',-1,'DataType',['unsigned int'],'ByteLayout',['little endian'],'SLDataType','SS_DOUBLE','Factor',1,'Offset',0),'StatusSelected','yes','TimeSelected','yes','DeltaTimeSelected','yes','BytePortSelected','no','MessageLengthSelected','no','EnablePortSelected','no','UserCoding',struct('Selected','no','InterfaceFile','UserDecodingFile','FcnName','UserDecodeFcn','InportSelected','no','InportWidth',1,'OutportSelected','no','OutportWidth',1),'TriggerPort',struct('Selected','no','TriggerType','rising'),'UseRXService','no','BoardType','DS4302','BoardNo',1,'ControllerNo',1,'SFcnPortType','Scalar'),'TLCFileName','rtican_rx_message')
      settings: AttributesFormatString=Group Id: RTICAN1\n  SourceProductName=dSPACE RTI CAN Blockset
  EEC3_00 : Outport
  wires:
  EEC3_001/3 -> Data Type Conversion8/1
  EEC3_001/4 -> Data Type Conversion9/1
  EEC3_001/5 -> Data Type Conversion10/1
  Enable/1 -> EEC3_001/Enable
  Bus Creator3/1 -> EEC3_00/1  "EEC3_00"
  EEC3_001/1 -> Data Type Conversion2/1  "SPN514_NominalFrictionPercentTorque"
  EEC3_001/2 -> Data Type Conversion1/1  "SPN2978_EstEngParasiticLossesPercentTorque"
  Data Type Conversion2/1 -> Bus Creator3/1  "SPN514_NominalFrictionPercentTorque"
  Data Type Conversion1/1 -> Bus Creator3/2  "SPN2978_EstEngParasiticLossesPercentTorque"
  Data Type Conversion8/1 -> Bus Creator3/3  "RX_status"
  Data Type Conversion9/1 -> Bus Creator3/4  "RX_time"
  Data Type Conversion10/1 -> Bus Creator3/5  "RX_delta_time"

== system SUB_ECU_L4_MABX_HW_Interface_PIC_KW/CAN_PIC_KW/CAN_RX_ETC2_03/RX_CAN_1 ==
  Enable : Inport
  Bus Creator3 : BusCreator  Inputs=6
  Data Type Conversion{1..3,9..10} (5 alike) : DataTypeConversion  OutDataTypeStr=double  SaturateOnIntegerOverflow=on
  Data Type Conversion8 : DataTypeConversion  OutDataTypeStr=boolean  SaturateOnIntegerOverflow=on
  ETC2_031 : rtican/RTICAN Receive (RX)   Reserved1=[]  Reserved2=[]  Reserved3=[]  Reserved4=[]  SfcnMessage=[]  Msg_Struct=[]  BoardTypeNo=[]  BoardNo=[]  ChannelNo=[]  Parameters=[]  DialogFcn=[]  UnitName=[]  Revision=[]  UnitValues=[]  DSProperties=struct('RTI',struct('Version',uint32(5),'BlockType',struct('isSLSource',uint8(1),'isSLSink',uint8(1),'isHWSource',uint8(0),'isHWSink',uint8(0),'isSetup',uint8(0),'isInline',uint8(1),'isNonInline',uint8(0),'isInterrupt',uint8(0),'isChannelwise',uint8(0)),'IOBoardType','RTICAN','UnitType','MESSAGE','Identifier','RX','DialogType','MSVC','BlockSet','RTICAN','SlaveProcessor','CAN'))  RTIBlockInterface=struct('OutputPortsWidth',int32([1 1 1 1 1 1]),'OutputPortsActive',[1 1 1 1 1 1],'OutputPortsName',{{'SPN524_TransSelectedGear','SPN526_TransActualGearRatio','SPN523_TransCurrentGear',['RX status'],['RX time'],['RX delta time']}},'OutputPortsDataType',{{'SS_DOUBLE','SS_DOUBLE','SS_DOUBLE','SS_DOUBLE','SS_DOUBLE','SS_DOUBLE'}},'OutputPortsLabel',{{'SPN524_TransSelectedGear','SPN526_TransActualGearRatio','SPN523_TransCurrentGear','','',''}},'OutputPortsLabelMode','ON','InputPortsWidth',int32(0),'InputPortsActive',0,'DialogFcn','rtican_message_interface_gui','BlockDisplay',{{'','center'}},'IconTransparency','on','ParameterTunableNames',{{}},'InitLevel',3,'BlockName',struct('Token',{{'ETC2_03'}}),'SampleTime',{{-1}},'TriggerPort',{{'none'}},'EnablePort',{{'yes'}})  RTIBlockParameters=struct('BoardTypeNo',{{1,'OFF',[]}},'BoardNo',{{1,'ON',[1 16]}},'ChannelNo',{{1,'ON',[1 2]}},'Parameters',{{struct('DataFileSupport',struct('DataFileSelectedMaster',1,'DataFileSelectedLocal',0,'DataFileName','i:\435\team\balton\truck1571\dbc\mabx_can1.dbc|','DataFileDate',{{{['01-Feb-2017 13:05:11']}}},'SelectedFile',['<no file selected>']),'Options',struct('StatusSelected',1,'TimeSelected',1,'DeltaTimeSelected',1,'BytePortSelected',0,'MessageLengthSelected',0,'TriggerPort',struct('Selected',0,'TriggerType',0),'UserCoding',struct('Selected',0,'InterfaceFile','UserDecodingFile','FcnName','UserDecodeFcn','InportSelected',0,'InportWidth',1,'OutportSelected',0,'OutportWidth',1),'EnablePortSelected',1,'SignalOnPortnameSelected',1,'UseRXService',1),'Message',struct('MsgOnBlocknameSelected',1,'MsgName','ETC2_03','MsgIdFormat',1,'MsgId',418383107,'MsgLength',8,'NumSignals',3,'SampleTime',-1,'Signal',struct('SgnName',{'SPN524_TransSelectedGear','SPN526_TransActualGearRatio','SPN523_TransCurrentGear'},'SgnStartBit',{0,8,24},'SgnLength',{8,16,8},'SgnType',{0,0,0},'ModeValue',{-1,-1,-1},'DataType',{0,0,0},'ByteLayout',{0,0,0},'Factor',{1,0.001,1},'Offset',{-125,0,-125},'SgnComment',{{''},{''},{''}},'SgnUnit',{'gear','ratio','gear'},'Min',{0,0,0},'Max',{0,0,0},'SLDataType',{'SS_DOUBLE','SS_DOUBLE','SS_DOUBLE'}),'MsgIdNumFormat',1,'MsgComment',{{['Electronic Transmission Controller 2']}}),'Version',1.2,'general',struct('isFromLib',0)),'OFF',[]}},'GroupId',{{struct('Group',{{'RTICAN'}},'No',1,'Behavior',{{'NAMECHANGE'}},'BlockType',{{'SINK'}},'NameChangeFlag',0),'OFF',[]}},'SFcnRTICANMessage',{{struct('MsgType','RX','SFcnPortType','Scalar','MsgName','ETC2_03','MsgIdFormat','XTD','MsgId',418383107,'MsgLength',8,'NumSignals',3,'SampleTime',-1,'Signal',struct('SgnName',{'SPN524_TransSelectedGear','SPN526_TransActualGearRatio','SPN523_TransCurrentGear'},'SgnStartBit',{0,8,24},'SgnLength',{8,16,8},'SgnType',{'standard','standard','standard'},'ModeValue',{-1,-1,-1},'DataType',{['unsigned int'],['unsigned int'],['unsigned int']},'ByteLayout',{['little endian'],['little endian'],['little endian']},'Factor',{1,0.001,1},'Offset',{-125,0,-125},'SLDataType',{'SS_DOUBLE','SS_DOUBLE','SS_DOUBLE'}),'StatusSelected','yes','TimeSelected','yes','DeltaTimeSelected','yes','BytePortSelected','no','MessageLengthSelected','no','TriggerPort',struct('Selected','no','TriggerType',0),'UserCoding',struct('Selected','no','InterfaceFile','UserDecodingFile','FcnName','UserDecodeFcn','InportSelected','no','InportWidth',1,'OutportSelected','no','OutportWidth',1),'EnablePortSelected','yes','UseRXService','yes','BoardType','DS1','BoardNo',1,'ControllerNo',2),'OFF',[]}},'TLCFileName',{{'rtican_rx_message','OFF',[]}})  RTISFcnParameters=struct('SFcnRTICANMessage','struct','TLCFileName','char')  RTIBlockParaDefault=struct('BoardTypeNo',4302,'BoardNo',1,'ChannelNo',1,'Parameters',struct('DataFileSupport',struct('DataFileSelectedMaster',0,'DataFileSelectedLocal',0,'DataFileName','','DataFileDate','','SelectedFile',['<no file selected>']),'Options',struct('StatusSelected',1,'TimeSelected',1,'DeltaTimeSelected',1,'BytePortSelected',0,'MessageLengthSelected',0,'TriggerPort',struct('Selected',0,'TriggerType','rising'),'UserCoding',struct('Selected',0,'InterfaceFile','UserDecodingFile','FcnName','UserDecodeFcn','InportSelected',0,'InportWidth',1,'OutportSelected',0,'OutportWidth',1),'EnablePortSelected',0,'SignalOnPortnameSelected',1,'UseRXService',0),'Message',struct('MsgOnBlocknameSelected',0,'MsgName',['RX Message'],'MsgIdFormat',0,'MsgId',100,'MsgLength',8,'NumSignals',1,'SampleTime',-1,'Signal',struct('SgnName',['RX signal'],'SgnStartBit',0,'SgnLength',8,'SgnType',0,'ModeValue',-1,'DataType',0,'SLDataType','SS_DOUBLE','ByteLayout',0,'Factor',1,'Offset',0,'Min',0,'Max',255,'SgnComment',{{}},'SgnUnit',''),'MsgIdNumFormat',0,'MsgComment',{{''}}),'Version',1.2,'general',struct('isFromLib',1)),'GroupId',struct('Group',{{'RTICAN'}},'No',1,'Behavior',{{'NAMECHANGE'}},'BlockType',{{'SINK'}},'NameChangeFlag',0),'SFcnRTICANMessage',struct('MsgType','RX','MsgName',['RX Message'],'MsgIdFormat','STD','MsgId',100,'MsgLength',8,'NumSignals',1,'SampleTime',-1,'Signal',struct('SgnName',['RX signal'],'SgnStartBit',0,'SgnLength',8,'SgnType','standard','ModeValue',-1,'DataType',['unsigned int'],'ByteLayout',['little endian'],'SLDataType','SS_DOUBLE','Factor',1,'Offset',0),'StatusSelected','yes','TimeSelected','yes','DeltaTimeSelected','yes','BytePortSelected','no','MessageLengthSelected','no','EnablePortSelected','no','UserCoding',struct('Selected','no','InterfaceFile','UserDecodingFile','FcnName','UserDecodeFcn','InportSelected','no','InportWidth',1,'OutportSelected','no','OutportWidth',1),'TriggerPort',struct('Selected','no','TriggerType','rising'),'UseRXService','no','BoardType','DS4302','BoardNo',1,'ControllerNo',1,'SFcnPortType','Scalar'),'TLCFileName','rtican_rx_message')
      settings: AttributesFormatString=Group Id: RTICAN1\n  SourceProductName=dSPACE RTI CAN Blockset
  ETC2_03 : Outport
  wires:
  Data Type Conversion9/1 -> Bus Creator3/5  "RX_time"
  Data Type Conversion10/1 -> Bus Creator3/6  "RX_delta_time"
  Data Type Conversion8/1 -> Bus Creator3/4  "RX_status"
  ETC2_031/4 -> Data Type Conversion8/1
  ETC2_031/5 -> Data Type Conversion9/1
  ETC2_031/6 -> Data Type Conversion10/1
  Enable/1 -> ETC2_031/Enable
  Bus Creator3/1 -> ETC2_03/1  "ETC2_03"
  ETC2_031/1 -> Data Type Conversion1/1
  ETC2_031/3 -> Data Type Conversion2/1
  Data Type Conversion1/1 -> Bus Creator3/1  "SPN524_TransSelectedGear"
  Data Type Conversion2/1 -> Bus Creator3/3  "SPN523_TransCurrentGear"
  ETC2_031/2 -> Data Type Conversion3/1
  Data Type Conversion3/1 -> Bus Creator3/2  "SPN526_TransActualGearRatio"
